simulink model "HW6_3"  (R2021a)
settings: Solver=VariableStepAuto  StartTime=0.0  StopTime=9  RelTol=1e-3
undefined symbols (not defined in the file or in its folder): w_fun
libraries: hdlBasic x207, simulink x2, xbsIndex_r4 x1
(part 1 of 2)
settings Model: Creator=hasith  LastModifiedBy=hasith

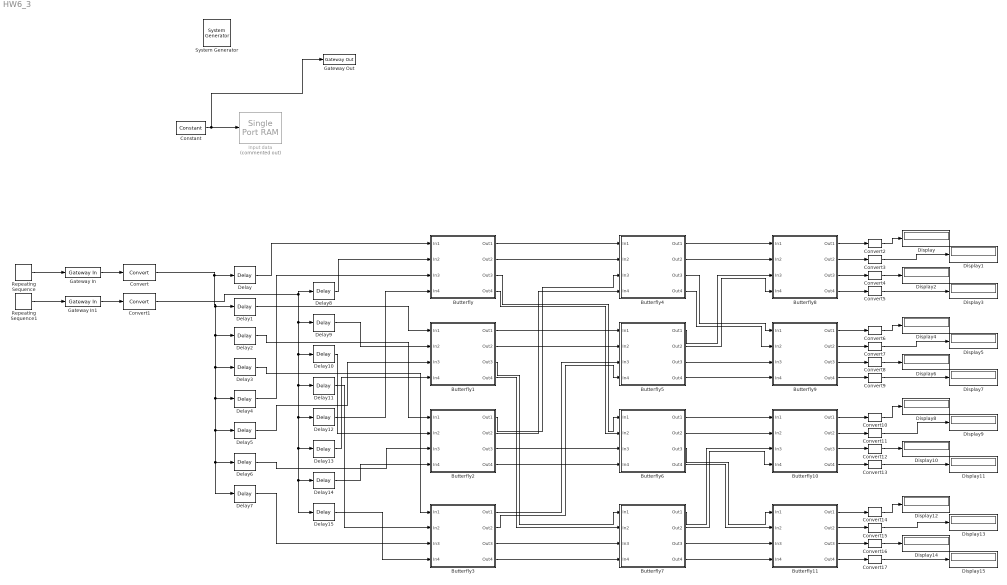
== system HW6_3 ==
  " System Generator" : xbsIndex_r4/ System Generator  Tag=genX  xilinxfamily=kintex7  part=xc7k325t  speed=-2  package=ffg900  synthesis_tool=Vivado  clock_wrapper=Clock Enables  directory=./netlist  proj_type=Vivado  Synth_file=Vivado Synthesis Defaults  Impl_file=Vivado Implementation Defaults  testbench=off  simulink_period=1  sysclk_period=10  dcm_input_clock_period=10  incr_netlist=off  trim_vbits=Everywhere in SubSystem  dbl_ovrd=According to Block Masks  core_generation=According to Block Masks  run_coregen=off  deprecated_control=off  eval_field=0  block_type=sysgen
  Butterfly : Subsystem  mask{wb_r=w_fun(0,8,1), wb_c=w_fun(0,8,1)}
      mask prompts: wb_r "w_r"; wb_c "w_c"
      mask Display:
      | port_label('input', 1, 'Re(x(n))')
      | port_label('input', 2, 'Im(x(n))')
      | port_label('input', 3, 'Re(x(n+N/2))')
      | port_label('input', 4, 'Im(x(n+N/2))')
      | 
      | 
      | port_label('output', 1, 'X_er')
      | port_label('output', 2, 'X_ei')
      | port_label('output', 3, 'X_or')
      | port_label('output',4, 'X_oi')
  Butterfly1 : Subsystem  mask{wb_r=w_fun(1,8,1), wb_c=w_fun(1,8,0)}
      mask prompts: wb_r "w_r"; wb_c "w_c"
      mask Display:
      | port_label('input', 1, 'Re(x(n))')
      | port_label('input', 2, 'Im(x(n))')
      | port_label('input', 3, 'Re(x(n+N/2))')
      | port_label('input', 4, 'Im(x(n+N/2))')
      | 
      | 
      | port_label('output', 1, 'X_er')
      | port_label('output', 2, 'X_ei')
      | port_label('output', 3, 'X_or')
      | port_label('output',4, 'X_oi')
  Butterfly10 : Subsystem  mask{wb_r=w_fun(0,8,1), wb_c=w_fun(0,8,0)}
      mask prompts: wb_r "w_r"; wb_c "w_c"
      mask Display:
      | port_label('input', 1, 'Re(x(n))')
      | port_label('input', 2, 'Im(x(n))')
      | port_label('input', 3, 'Re(x(n+N/2))')
      | port_label('input', 4, 'Im(x(n+N/2))')
      | 
      | 
      | port_label('output', 1, 'X_er')
      | port_label('output', 2, 'X_ei')
      | port_label('output', 3, 'X_or')
      | port_label('output',4, 'X_oi')
  Butterfly11 : Subsystem  mask{wb_r=w_fun(0,8,1), wb_c=w_fun(0,8,0)}
      mask prompts: wb_r "w_r"; wb_c "w_c"
      mask Display:
      | port_label('input', 1, 'Re(x(n))')
      | port_label('input', 2, 'Im(x(n))')
      | port_label('input', 3, 'Re(x(n+N/2))')
      | port_label('input', 4, 'Im(x(n+N/2))')
      | 
      | 
      | port_label('output', 1, 'X_er')
      | port_label('output', 2, 'X_ei')
      | port_label('output', 3, 'X_or')
      | port_label('output',4, 'X_oi')
  Butterfly2 : Subsystem  mask{wb_r=w_fun(2,8,1), wb_c=w_fun(2,8,0)}
      mask prompts: wb_r "w_r"; wb_c "w_c"
      mask Display:
      | port_label('input', 1, 'Re(x(n))')
      | port_label('input', 2, 'Im(x(n))')
      | port_label('input', 3, 'Re(x(n+N/2))')
      | port_label('input', 4, 'Im(x(n+N/2))')
      | 
      | 
      | port_label('output', 1, 'X_er')
      | port_label('output', 2, 'X_ei')
      | port_label('output', 3, 'X_or')
      | port_label('output',4, 'X_oi')
  Butterfly3 : Subsystem  mask{wb_r=w_fun(3,8,1), wb_c=w_fun(3,8,0)}
      mask prompts: wb_r "w_r"; wb_c "w_c"
      mask Display:
      | port_label('input', 1, 'Re(x(n))')
      | port_label('input', 2, 'Im(x(n))')
      | port_label('input', 3, 'Re(x(n+N/2))')
      | port_label('input', 4, 'Im(x(n+N/2))')
      | 
      | 
      | port_label('output', 1, 'X_er')
      | port_label('output', 2, 'X_ei')
      | port_label('output', 3, 'X_or')
      | port_label('output',4, 'X_oi')
  Butterfly4 : Subsystem  mask{wb_r=w_fun(0,8,1), wb_c=w_fun(0,8,0)}
      mask prompts: wb_r "w_r"; wb_c "w_c"
      mask Display:
      | port_label('input', 1, 'Re(x(n))')
      | port_label('input', 2, 'Im(x(n))')
      | port_label('input', 3, 'Re(x(n+N/2))')
      | port_label('input', 4, 'Im(x(n+N/2))')
      | 
      | 
      | port_label('output', 1, 'X_er')
      | port_label('output', 2, 'X_ei')
      | port_label('output', 3, 'X_or')
      | port_label('output',4, 'X_oi')
  Butterfly5 : Subsystem  mask{wb_r=w_fun(2,8,1), wb_c=w_fun(2,8,0)}
      mask prompts: wb_r "w_r"; wb_c "w_c"
      mask Display:
      | port_label('input', 1, 'Re(x(n))')
      | port_label('input', 2, 'Im(x(n))')
      | port_label('input', 3, 'Re(x(n+N/2))')
      | port_label('input', 4, 'Im(x(n+N/2))')
      | 
      | 
      | port_label('output', 1, 'X_er')
      | port_label('output', 2, 'X_ei')
      | port_label('output', 3, 'X_or')
      | port_label('output',4, 'X_oi')
  Butterfly6 : Subsystem  mask{wb_r=w_fun(0,8,1), wb_c=w_fun(0,8,0)}
      mask prompts: wb_r "w_r"; wb_c "w_c"
      mask Display:
      | port_label('input', 1, 'Re(x(n))')
      | port_label('input', 2, 'Im(x(n))')
      | port_label('input', 3, 'Re(x(n+N/2))')
      | port_label('input', 4, 'Im(x(n+N/2))')
      | 
      | 
      | port_label('output', 1, 'X_er')
      | port_label('output', 2, 'X_ei')
      | port_label('output', 3, 'X_or')
      | port_label('output',4, 'X_oi')
  Butterfly7 : Subsystem  mask{wb_r=w_fun(2,8,1), wb_c=w_fun(2,8,0)}
      mask prompts: wb_r "w_r"; wb_c "w_c"
      mask Display:
      | port_label('input', 1, 'Re(x(n))')
      | port_label('input', 2, 'Im(x(n))')
      | port_label('input', 3, 'Re(x(n+N/2))')
      | port_label('input', 4, 'Im(x(n+N/2))')
      | 
      | 
      | port_label('output', 1, 'X_er')
      | port_label('output', 2, 'X_ei')
      | port_label('output', 3, 'X_or')
      | port_label('output',4, 'X_oi')
  Butterfly8 : Subsystem  mask{wb_r=w_fun(0,8,1), wb_c=w_fun(0,8,0)}
      mask prompts: wb_r "w_r"; wb_c "w_c"
      mask Display:
      | port_label('input', 1, 'Re(x(n))')
      | port_label('input', 2, 'Im(x(n))')
      | port_label('input', 3, 'Re(x(n+N/2))')
      | port_label('input', 4, 'Im(x(n+N/2))')
      | 
      | 
      | port_label('output', 1, 'X_er')
      | port_label('output', 2, 'X_ei')
      | port_label('output', 3, 'X_or')
      | port_label('output',4, 'X_oi')
  Butterfly9 : Subsystem  mask{wb_r=w_fun(0,8,1), wb_c=w_fun(0,8,0)}
      mask prompts: wb_r "w_r"; wb_c "w_c"
      mask Display:
      | port_label('input', 1, 'Re(x(n))')
      | port_label('input', 2, 'Im(x(n))')
      | port_label('input', 3, 'Re(x(n+N/2))')
      | port_label('input', 4, 'Im(x(n+N/2))')
      | 
      | 
      | port_label('output', 1, 'X_er')
      | port_label('output', 2, 'X_ei')
      | port_label('output', 3, 'X_or')
      | port_label('output',4, 'X_oi')
  Constant : hdlBasic/Constant  const=0  gui_display_data_type=Fixed-point  arith_type=Signed (2's comp)  n_bits=8  bin_pt=0  preci_type=Custom  exp_width=9  frac_width=9  explicit_period=off  period=1  XmcBlockStatus=1  maskContainerNames=tabcontainer1  block_type=constant  block_config=sysgen:Constant_config
  Convert : hdlBasic/Convert  gui_display_data_type=Floating-point  arith_type=Floating-point  n_bits=16  bin_pt=14  float_type=Custom  exp_bits=9  fraction_bits=9  quantization=Truncate  overflow=Wrap  en=off  latency=0  pipeline=off  XmcBlockStatus=1  maskContainerNames=group2  block_type=convert  block_config=sysgen:Convert_config
  Convert1 : hdlBasic/Convert  gui_display_data_type=Floating-point  arith_type=Floating-point  n_bits=16  bin_pt=14  float_type=Custom  exp_bits=9  fraction_bits=9  quantization=Truncate  overflow=Wrap  en=off  latency=0  pipeline=off  XmcBlockStatus=1  maskContainerNames=group2  block_type=convert  block_config=sysgen:Convert_config
  Convert{2..17} (16 alike) : hdlBasic/Convert  gui_display_data_type=Floating-point  arith_type=Floating-point  n_bits=16  bin_pt=14  float_type=Single  exp_bits=9  fraction_bits=9  quantization=Truncate  overflow=Wrap  en=off  latency=0  pipeline=off  XmcBlockStatus=1  maskContainerNames=group2  block_type=convert  block_config=sysgen:Convert_config
  Delay : hdlBasic/Delay  rst=off  en=off  latency=1  reg_retiming=off  XmcBlockStatus=1  maskContainerNames=group1  block_type=delay  block_config=sysgen:Delay_config
  Delay1 : hdlBasic/Delay  rst=off  en=off  latency=2  reg_retiming=off  XmcBlockStatus=1  maskContainerNames=group1  block_type=delay  block_config=sysgen:Delay_config
  Delay10 : hdlBasic/Delay  rst=off  en=off  latency=3  reg_retiming=off  XmcBlockStatus=1  maskContainerNames=group1  block_type=delay  block_config=sysgen:Delay_config
  Delay11 : hdlBasic/Delay  rst=off  en=off  latency=4  reg_retiming=off  XmcBlockStatus=1  maskContainerNames=group1  block_type=delay  block_config=sysgen:Delay_config
  Delay12 : hdlBasic/Delay  rst=off  en=off  latency=5  reg_retiming=off  XmcBlockStatus=1  maskContainerNames=group1  block_type=delay  block_config=sysgen:Delay_config
  Delay13 : hdlBasic/Delay  rst=off  en=off  latency=6  reg_retiming=off  XmcBlockStatus=1  maskContainerNames=group1  block_type=delay  block_config=sysgen:Delay_config
  Delay14 : hdlBasic/Delay  rst=off  en=off  latency=7  reg_retiming=off  XmcBlockStatus=1  maskContainerNames=group1  block_type=delay  block_config=sysgen:Delay_config
  Delay15 : hdlBasic/Delay  rst=off  en=off  latency=8  reg_retiming=off  XmcBlockStatus=1  maskContainerNames=group1  block_type=delay  block_config=sysgen:Delay_config
  Delay2 : hdlBasic/Delay  rst=off  en=off  latency=3  reg_retiming=off  XmcBlockStatus=1  maskContainerNames=group1  block_type=delay  block_config=sysgen:Delay_config
  Delay3 : hdlBasic/Delay  rst=off  en=off  latency=4  reg_retiming=off  XmcBlockStatus=1  maskContainerNames=group1  block_type=delay  block_config=sysgen:Delay_config
  Delay4 : hdlBasic/Delay  rst=off  en=off  latency=5  reg_retiming=off  XmcBlockStatus=1  maskContainerNames=group1  block_type=delay  block_config=sysgen:Delay_config
  Delay5 : hdlBasic/Delay  rst=off  en=off  latency=6  reg_retiming=off  XmcBlockStatus=1  maskContainerNames=group1  block_type=delay  block_config=sysgen:Delay_config
  Delay6 : hdlBasic/Delay  rst=off  en=off  latency=7  reg_retiming=off  XmcBlockStatus=1  maskContainerNames=group1  block_type=delay  block_config=sysgen:Delay_config
  Delay7 : hdlBasic/Delay  rst=off  en=off  latency=8  reg_retiming=off  XmcBlockStatus=1  maskContainerNames=group1  block_type=delay  block_config=sysgen:Delay_config
  Delay8 : hdlBasic/Delay  rst=off  en=off  latency=1  reg_retiming=off  XmcBlockStatus=1  maskContainerNames=group1  block_type=delay  block_config=sysgen:Delay_config
  Delay9 : hdlBasic/Delay  rst=off  en=off  latency=2  reg_retiming=off  XmcBlockStatus=1  maskContainerNames=group1  block_type=delay  block_config=sysgen:Delay_config
  Display{,1..15} (16 alike) : Display
  Gateway In : hdlBasic/Gateway In  gui_display_data_type=Floating-point  arith_type=Floating-point  n_bits=8  bin_pt=0  preci_type=Single  exp_width=8  frac_width=24  rows=1  columns=1  quantization=Truncate  overflow=Saturate  period=1  UseAsADC=off  ADCChannel='1'  interface=None  automatic_assignment=on  address_offset=hex2dec('00')  intf_name=''  intf_description=''  default_value=0  timing_constraint=None  locs_specified=off  LOCs={}  io_standard={}  inherit_from_input=off  hdl_port=on  XmcBlockStatus=1  maskContainerNames=group4  block_type=gatewayin  block_config=sysgen:gateway_in_config  block_width_w=590  block_height_w=620  block_width=640  block_height=850
  Gateway In1 : hdlBasic/Gateway In  gui_display_data_type=Floating-point  arith_type=Floating-point  n_bits=8  bin_pt=0  preci_type=Single  exp_width=8  frac_width=24  rows=1  columns=1  quantization=Truncate  overflow=Saturate  period=1  UseAsADC=off  ADCChannel='1'  interface=None  automatic_assignment=on  address_offset=hex2dec('00')  intf_name=''  intf_description=''  default_value=0  timing_constraint=None  locs_specified=off  LOCs={}  io_standard={}  inherit_from_input=off  hdl_port=on  XmcBlockStatus=1  maskContainerNames=group4  block_type=gatewayin  block_config=sysgen:gateway_in_config  block_width_w=590  block_height_w=620  block_width=640  block_height=850
  Gateway Out : hdlBasic/Gateway Out  inherit_from_input=off  hdl_port=on  rows=1  columns=1  UseAsDAC=off  DACChannel='1'  interface=None  automatic_assignment=on  address_offset=hex2dec('00')  intf_name=''  intf_description=''  timing_constraint=None  locs_specified=off  LOCs={}  io_standard={}  XmcBlockStatus=1  maskContainerNames=group4  block_type=gatewayout  block_config=sysgen:gateway_out_config  block_width_w=590  block_height_w=620  block_width=620  block_height=750
  Input data : hdlBasic/Single Port RAM  Commented=on  depth=N  initVector=y  distributed_mem=Block RAM  write_mode=No Read On Write  rst=off  init_reg=0  en=off  optimize_latency=off  latency=1  optimize=Area  dbl_ovrd=off  simulation_type=fast_sim  XmcBlockStatus=1  maskContainerNames=tabcontainer1  block_type=spram  block_config=sysgen:SPRAM_config
  Repeating Sequence : simulink/Sources/Repeating Sequence  rep_seq_t=0:8  rep_seq_y=0:8
  Repeating Sequence1 : simulink/Sources/Repeating Sequence  rep_seq_t=0:8  rep_seq_y=[0 0 0 0 0 0 0 0 0]
  wires:
  Constant/1 -> Gateway Out/1, Input data/2
  Repeating Sequence/1 -> Gateway In/1
  Gateway In/1 -> Convert/1
  Gateway In1/1 -> Convert1/1
  Repeating Sequence1/1 -> Gateway In1/1
  Delay/1 -> Butterfly/1(In1)
  Delay8/1 -> Butterfly/2(In2)
  Delay4/1 -> Butterfly/3(In3)
  Delay12/1 -> Butterfly/4(In4)
  Delay9/1 -> Butterfly1/2(In2)
  Delay1/1 -> Butterfly1/1(In1)
  Delay5/1 -> Butterfly1/3(In3)
  Delay13/1 -> Butterfly1/4(In4)
  Delay2/1 -> Butterfly2/1(In1)
  Delay10/1 -> Butterfly2/2(In2)
  Delay6/1 -> Butterfly2/3(In3)
  Delay14/1 -> Butterfly2/4(In4)
  Delay3/1 -> Butterfly3/1(In1)
  Delay7/1 -> Butterfly3/3(In3)
  Delay11/1 -> Butterfly3/2(In2)
  Delay15/1 -> Butterfly3/4(In4)
  Butterfly/1(Out1) -> Butterfly4/1(In1)
  Butterfly/2(Out2) -> Butterfly4/2(In2)
  Butterfly2/1(Out1) -> Butterfly4/3(In3)
  Butterfly2/2(Out2) -> Butterfly4/4(In4)
  Butterfly1/1(Out1) -> Butterfly5/1(In1)
  Butterfly1/2(Out2) -> Butterfly5/2(In2)
  Butterfly3/1(Out1) -> Butterfly5/3(In3)
  Butterfly3/2(Out2) -> Butterfly5/4(In4)
  Butterfly/3(Out3) -> Butterfly6/1(In1)
  Butterfly/4(Out4) -> Butterfly6/2(In2)
  Butterfly2/3(Out3) -> Butterfly6/3(In3)
  Butterfly2/4(Out4) -> Butterfly6/4(In4)
  Butterfly1/3(Out3) -> Butterfly7/1(In1)
  Butterfly1/4(Out4) -> Butterfly7/2(In2)
  Butterfly3/3(Out3) -> Butterfly7/3(In3)
  Butterfly3/4(Out4) -> Butterfly7/4(In4)
  Butterfly4/1(Out1) -> Butterfly8/1(In1)
  Butterfly4/2(Out2) -> Butterfly8/2(In2)
  Butterfly5/1(Out1) -> Butterfly8/3(In3)
  Butterfly5/2(Out2) -> Butterfly8/4(In4)
  Butterfly4/3(Out3) -> Butterfly9/1(In1)
  Butterfly4/4(Out4) -> Butterfly9/2(In2)
  Butterfly5/3(Out3) -> Butterfly9/3(In3)
  Butterfly5/4(Out4) -> Butterfly9/4(In4)
  Butterfly6/1(Out1) -> Butterfly10/1(In1)
  Butterfly6/2(Out2) -> Butterfly10/2(In2)
  Butterfly7/4(Out4) -> Butterfly11/4(In4)
  Butterfly7/3(Out3) -> Butterfly11/3(In3)
  Butterfly6/3(Out3) -> Butterfly11/1(In1)
  Butterfly6/4(Out4) -> Butterfly11/2(In2)
  Butterfly7/1(Out1) -> Butterfly10/3(In3)
  Butterfly7/2(Out2) -> Butterfly10/4(In4)
  Convert/1 -> Delay2/1, Delay7/1, Delay6/1, Delay5/1, Delay4/1, Delay3/1, Delay1/1, Delay/1
  Convert1/1 -> Delay8/1, Delay11/1, Delay12/1, Delay15/1, Delay14/1, Delay13/1, Delay10/1, Delay9/1
  Butterfly8/1(Out1) -> Convert2/1
  Butterfly8/2(Out2) -> Convert3/1
  Butterfly8/3(Out3) -> Convert4/1
  Butterfly8/4(Out4) -> Convert5/1
  Convert2/1 -> Display/1
  Convert3/1 -> Display1/1
  Convert4/1 -> Display2/1
  Convert5/1 -> Display3/1
  Butterfly9/1(Out1) -> Convert6/1
  Butterfly9/2(Out2) -> Convert7/1
  Butterfly9/4(Out4) -> Convert9/1
  Convert6/1 -> Display4/1
  Butterfly9/3(Out3) -> Convert8/1
  Convert7/1 -> Display5/1
  Convert8/1 -> Display6/1
  Convert9/1 -> Display7/1
  Butterfly10/1(Out1) -> Convert10/1
  Butterfly10/2(Out2) -> Convert11/1
  Butterfly10/4(Out4) -> Convert13/1
  Convert10/1 -> Display8/1
  Butterfly10/3(Out3) -> Convert12/1
  Convert11/1 -> Display9/1
  Convert12/1 -> Display10/1
  Convert13/1 -> Display11/1
  Butterfly11/1(Out1) -> Convert14/1
  Butterfly11/2(Out2) -> Convert15/1
  Butterfly11/4(Out4) -> Convert17/1
  Convert14/1 -> Display12/1
  Butterfly11/3(Out3) -> Convert16/1
  Convert15/1 -> Display13/1
  Convert16/1 -> Display14/1
  Convert17/1 -> Display15/1

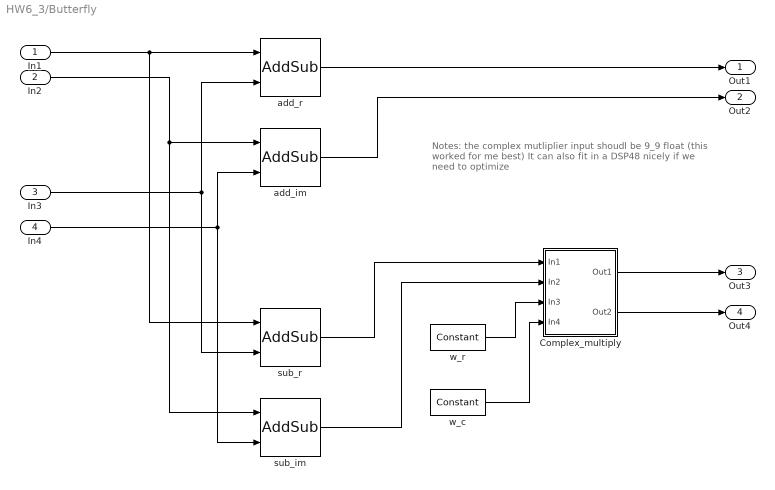
== system HW6_3/Butterfly ==
  note: Notes: the complex mutliplier
      | input shoudl be 9_9 float (this worked for me best)
      | It can also fit in a DSP48 nicely if we need to optimize
  In1 : Inport
  In2 : Inport  Port=2
  In3 : Inport  Port=3
  In4 : Inport  Port=4
  Complex_multiply : Subsystem
      mask Display:
      | port_label('input', 1, 'A')
      | port_label('input', 2, 'B')
      | port_label('input', 3, 'C')
      | port_label('input', 4, 'D')
      | 
      | 
      | port_label('output', 1, 'Real')
      | port_label('output', 2, 'Imag')
  add_im : hdlBasic/AddSub  mode=Addition  use_carryin=off  use_carryout=off  en=off  latency=0  precision=Full  arith_type=Unsigned  n_bits=16  bin_pt=14  quantization=Truncate  overflow=Wrap  use_behavioral_HDL=off  hw_selection=Fabric  pipelined=off  XmcBlockStatus=1  maskContainerNames=tabcontainer1  block_type=addsub  block_config=sysgen:Addsub_config
  add_r : hdlBasic/AddSub  mode=Addition  use_carryin=off  use_carryout=off  en=off  latency=0  precision=Full  arith_type=Unsigned  n_bits=16  bin_pt=14  quantization=Truncate  overflow=Wrap  use_behavioral_HDL=off  hw_selection=Fabric  pipelined=off  XmcBlockStatus=1  maskContainerNames=tabcontainer1  block_type=addsub  block_config=sysgen:Addsub_config
  sub_im : hdlBasic/AddSub  mode=Subtraction  use_carryin=off  use_carryout=off  en=off  latency=0  precision=Full  arith_type=Unsigned  n_bits=16  bin_pt=14  quantization=Truncate  overflow=Wrap  use_behavioral_HDL=off  hw_selection=Fabric  pipelined=off  XmcBlockStatus=1  maskContainerNames=tabcontainer1  block_type=addsub  block_config=sysgen:Addsub_config
  sub_r : hdlBasic/AddSub  mode=Subtraction  use_carryin=off  use_carryout=off  en=off  latency=0  precision=Full  arith_type=Unsigned  n_bits=16  bin_pt=14  quantization=Truncate  overflow=Wrap  use_behavioral_HDL=off  hw_selection=Fabric  pipelined=off  XmcBlockStatus=1  maskContainerNames=tabcontainer1  block_type=addsub  block_config=sysgen:Addsub_config
  w_c : hdlBasic/Constant  const=wb_c  gui_display_data_type=Floating-point  arith_type=Floating-point  n_bits=16  bin_pt=14  preci_type=Custom  exp_width=9  frac_width=9  explicit_period=off  period=1  XmcBlockStatus=1  maskContainerNames=tabcontainer1  block_type=constant  block_config=sysgen:Constant_config
  w_r : hdlBasic/Constant  const=wb_r  gui_display_data_type=Floating-point  arith_type=Floating-point  n_bits=16  bin_pt=14  preci_type=Custom  exp_width=9  frac_width=9  explicit_period=off  period=1  XmcBlockStatus=1  maskContainerNames=tabcontainer1  block_type=constant  block_config=sysgen:Constant_config
  Out1 : Outport
  Out2 : Outport  Port=2
  Out3 : Outport  Port=3
  Out4 : Outport  Port=4
  wires:
  Complex_multiply/2(Out2) -> Out4/1
  add_im/1 -> Out2/1
  w_r/1 -> Complex_multiply/3(In3)
  sub_r/1 -> Complex_multiply/1(In1)
  Complex_multiply/1(Out1) -> Out3/1
  In4/1 -> add_im/2, sub_im/2
  In3/1 -> add_r/2, sub_r/2
  add_r/1 -> Out1/1
  w_c/1 -> Complex_multiply/4(In4)
  sub_im/1 -> Complex_multiply/2(In2)
  In2/1 -> sub_im/1, add_im/1
  In1/1 -> sub_r/1, add_r/1

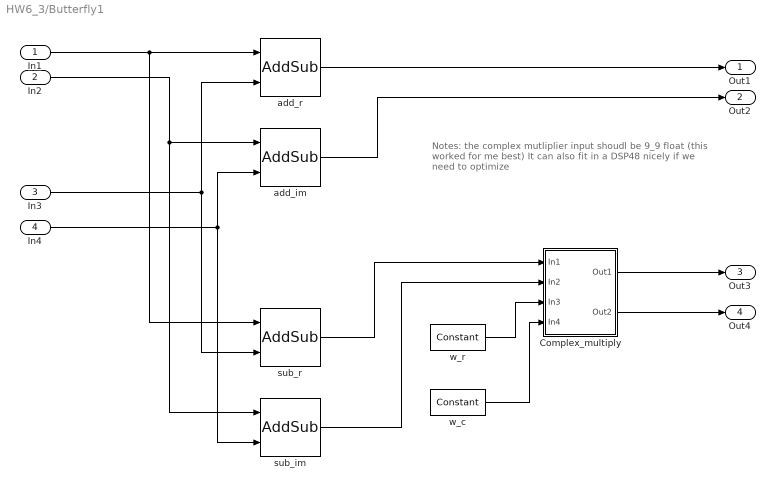
== system HW6_3/Butterfly1 ==
  note: Notes: the complex mutliplier
      | input shoudl be 9_9 float (this worked for me best)
      | It can also fit in a DSP48 nicely if we need to optimize
  In1 : Inport
  In2 : Inport  Port=2
  In3 : Inport  Port=3
  In4 : Inport  Port=4
  Complex_multiply : Subsystem
      mask Display:
      | port_label('input', 1, 'A')
      | port_label('input', 2, 'B')
      | port_label('input', 3, 'C')
      | port_label('input', 4, 'D')
      | 
      | 
      | port_label('output', 1, 'Real')
      | port_label('output', 2, 'Imag')
  add_im : hdlBasic/AddSub  mode=Addition  use_carryin=off  use_carryout=off  en=off  latency=0  precision=Full  arith_type=Unsigned  n_bits=16  bin_pt=14  quantization=Truncate  overflow=Wrap  use_behavioral_HDL=off  hw_selection=Fabric  pipelined=off  XmcBlockStatus=1  maskContainerNames=tabcontainer1  block_type=addsub  block_config=sysgen:Addsub_config
  add_r : hdlBasic/AddSub  mode=Addition  use_carryin=off  use_carryout=off  en=off  latency=0  precision=Full  arith_type=Unsigned  n_bits=16  bin_pt=14  quantization=Truncate  overflow=Wrap  use_behavioral_HDL=off  hw_selection=Fabric  pipelined=off  XmcBlockStatus=1  maskContainerNames=tabcontainer1  block_type=addsub  block_config=sysgen:Addsub_config
  sub_im : hdlBasic/AddSub  mode=Subtraction  use_carryin=off  use_carryout=off  en=off  latency=0  precision=Full  arith_type=Unsigned  n_bits=16  bin_pt=14  quantization=Truncate  overflow=Wrap  use_behavioral_HDL=off  hw_selection=Fabric  pipelined=off  XmcBlockStatus=1  maskContainerNames=tabcontainer1  block_type=addsub  block_config=sysgen:Addsub_config
  sub_r : hdlBasic/AddSub  mode=Subtraction  use_carryin=off  use_carryout=off  en=off  latency=0  precision=Full  arith_type=Unsigned  n_bits=16  bin_pt=14  quantization=Truncate  overflow=Wrap  use_behavioral_HDL=off  hw_selection=Fabric  pipelined=off  XmcBlockStatus=1  maskContainerNames=tabcontainer1  block_type=addsub  block_config=sysgen:Addsub_config
  w_c : hdlBasic/Constant  const=wb_c  gui_display_data_type=Floating-point  arith_type=Floating-point  n_bits=16  bin_pt=14  preci_type=Custom  exp_width=9  frac_width=9  explicit_period=off  period=1  XmcBlockStatus=1  maskContainerNames=tabcontainer1  block_type=constant  block_config=sysgen:Constant_config
  w_r : hdlBasic/Constant  const=wb_r  gui_display_data_type=Floating-point  arith_type=Floating-point  n_bits=16  bin_pt=14  preci_type=Custom  exp_width=9  frac_width=9  explicit_period=off  period=1  XmcBlockStatus=1  maskContainerNames=tabcontainer1  block_type=constant  block_config=sysgen:Constant_config
  Out1 : Outport
  Out2 : Outport  Port=2
  Out3 : Outport  Port=3
  Out4 : Outport  Port=4
  wires:
  Complex_multiply/2(Out2) -> Out4/1
  add_im/1 -> Out2/1
  w_r/1 -> Complex_multiply/3(In3)
  sub_r/1 -> Complex_multiply/1(In1)
  Complex_multiply/1(Out1) -> Out3/1
  In4/1 -> add_im/2, sub_im/2
  In3/1 -> add_r/2, sub_r/2
  add_r/1 -> Out1/1
  w_c/1 -> Complex_multiply/4(In4)
  sub_im/1 -> Complex_multiply/2(In2)
  In2/1 -> sub_im/1, add_im/1
  In1/1 -> sub_r/1, add_r/1

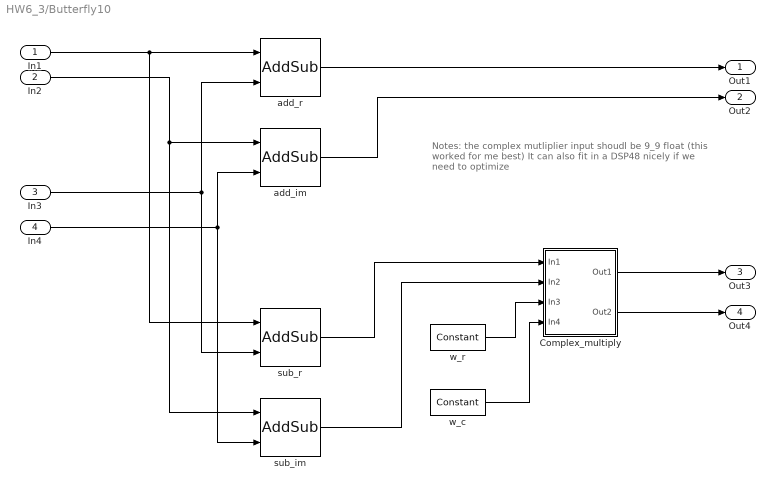
== system HW6_3/Butterfly10 ==
  note: Notes: the complex mutliplier
      | input shoudl be 9_9 float (this worked for me best)
      | It can also fit in a DSP48 nicely if we need to optimize
  In1 : Inport
  In2 : Inport  Port=2
  In3 : Inport  Port=3
  In4 : Inport  Port=4
  Complex_multiply : Subsystem
      mask Display:
      | port_label('input', 1, 'A')
      | port_label('input', 2, 'B')
      | port_label('input', 3, 'C')
      | port_label('input', 4, 'D')
      | 
      | 
      | port_label('output', 1, 'Real')
      | port_label('output', 2, 'Imag')
  add_im : hdlBasic/AddSub  mode=Addition  use_carryin=off  use_carryout=off  en=off  latency=0  precision=Full  arith_type=Unsigned  n_bits=16  bin_pt=14  quantization=Truncate  overflow=Wrap  use_behavioral_HDL=off  hw_selection=Fabric  pipelined=off  XmcBlockStatus=1  maskContainerNames=tabcontainer1  block_type=addsub  block_config=sysgen:Addsub_config
  add_r : hdlBasic/AddSub  mode=Addition  use_carryin=off  use_carryout=off  en=off  latency=0  precision=Full  arith_type=Unsigned  n_bits=16  bin_pt=14  quantization=Truncate  overflow=Wrap  use_behavioral_HDL=off  hw_selection=Fabric  pipelined=off  XmcBlockStatus=1  maskContainerNames=tabcontainer1  block_type=addsub  block_config=sysgen:Addsub_config
  sub_im : hdlBasic/AddSub  mode=Subtraction  use_carryin=off  use_carryout=off  en=off  latency=0  precision=Full  arith_type=Unsigned  n_bits=16  bin_pt=14  quantization=Truncate  overflow=Wrap  use_behavioral_HDL=off  hw_selection=Fabric  pipelined=off  XmcBlockStatus=1  maskContainerNames=tabcontainer1  block_type=addsub  block_config=sysgen:Addsub_config
  sub_r : hdlBasic/AddSub  mode=Subtraction  use_carryin=off  use_carryout=off  en=off  latency=0  precision=Full  arith_type=Unsigned  n_bits=16  bin_pt=14  quantization=Truncate  overflow=Wrap  use_behavioral_HDL=off  hw_selection=Fabric  pipelined=off  XmcBlockStatus=1  maskContainerNames=tabcontainer1  block_type=addsub  block_config=sysgen:Addsub_config
  w_c : hdlBasic/Constant  const=wb_c  gui_display_data_type=Floating-point  arith_type=Floating-point  n_bits=16  bin_pt=14  preci_type=Custom  exp_width=9  frac_width=9  explicit_period=off  period=1  XmcBlockStatus=1  maskContainerNames=tabcontainer1  block_type=constant  block_config=sysgen:Constant_config
  w_r : hdlBasic/Constant  const=wb_r  gui_display_data_type=Floating-point  arith_type=Floating-point  n_bits=16  bin_pt=14  preci_type=Custom  exp_width=9  frac_width=9  explicit_period=off  period=1  XmcBlockStatus=1  maskContainerNames=tabcontainer1  block_type=constant  block_config=sysgen:Constant_config
  Out1 : Outport
  Out2 : Outport  Port=2
  Out3 : Outport  Port=3
  Out4 : Outport  Port=4
  wires:
  Complex_multiply/2(Out2) -> Out4/1
  add_im/1 -> Out2/1
  w_r/1 -> Complex_multiply/3(In3)
  sub_r/1 -> Complex_multiply/1(In1)
  Complex_multiply/1(Out1) -> Out3/1
  In4/1 -> add_im/2, sub_im/2
  In3/1 -> add_r/2, sub_r/2
  add_r/1 -> Out1/1
  w_c/1 -> Complex_multiply/4(In4)
  sub_im/1 -> Complex_multiply/2(In2)
  In2/1 -> sub_im/1, add_im/1
  In1/1 -> sub_r/1, add_r/1

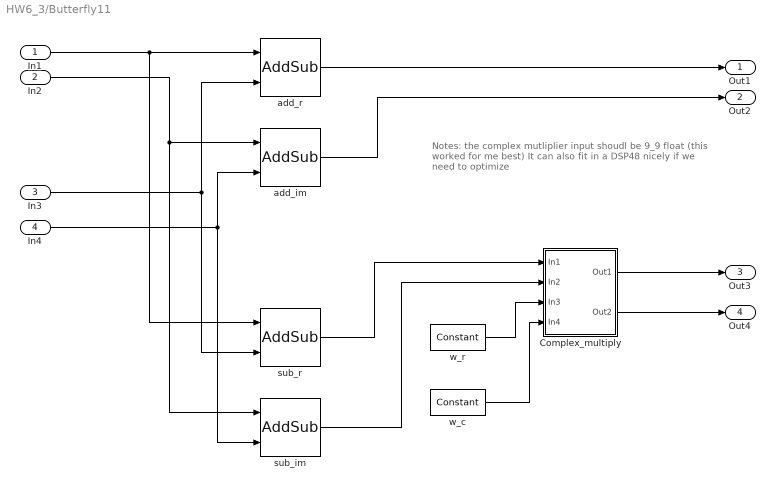
== system HW6_3/Butterfly11 ==
  note: Notes: the complex mutliplier
      | input shoudl be 9_9 float (this worked for me best)
      | It can also fit in a DSP48 nicely if we need to optimize
  In1 : Inport
  In2 : Inport  Port=2
  In3 : Inport  Port=3
  In4 : Inport  Port=4
  Complex_multiply : Subsystem
      mask Display:
      | port_label('input', 1, 'A')
      | port_label('input', 2, 'B')
      | port_label('input', 3, 'C')
      | port_label('input', 4, 'D')
      | 
      | 
      | port_label('output', 1, 'Real')
      | port_label('output', 2, 'Imag')
  add_im : hdlBasic/AddSub  mode=Addition  use_carryin=off  use_carryout=off  en=off  latency=0  precision=Full  arith_type=Unsigned  n_bits=16  bin_pt=14  quantization=Truncate  overflow=Wrap  use_behavioral_HDL=off  hw_selection=Fabric  pipelined=off  XmcBlockStatus=1  maskContainerNames=tabcontainer1  block_type=addsub  block_config=sysgen:Addsub_config
  add_r : hdlBasic/AddSub  mode=Addition  use_carryin=off  use_carryout=off  en=off  latency=0  precision=Full  arith_type=Unsigned  n_bits=16  bin_pt=14  quantization=Truncate  overflow=Wrap  use_behavioral_HDL=off  hw_selection=Fabric  pipelined=off  XmcBlockStatus=1  maskContainerNames=tabcontainer1  block_type=addsub  block_config=sysgen:Addsub_config
  sub_im : hdlBasic/AddSub  mode=Subtraction  use_carryin=off  use_carryout=off  en=off  latency=0  precision=Full  arith_type=Unsigned  n_bits=16  bin_pt=14  quantization=Truncate  overflow=Wrap  use_behavioral_HDL=off  hw_selection=Fabric  pipelined=off  XmcBlockStatus=1  maskContainerNames=tabcontainer1  block_type=addsub  block_config=sysgen:Addsub_config
  sub_r : hdlBasic/AddSub  mode=Subtraction  use_carryin=off  use_carryout=off  en=off  latency=0  precision=Full  arith_type=Unsigned  n_bits=16  bin_pt=14  quantization=Truncate  overflow=Wrap  use_behavioral_HDL=off  hw_selection=Fabric  pipelined=off  XmcBlockStatus=1  maskContainerNames=tabcontainer1  block_type=addsub  block_config=sysgen:Addsub_config
  w_c : hdlBasic/Constant  const=wb_c  gui_display_data_type=Floating-point  arith_type=Floating-point  n_bits=16  bin_pt=14  preci_type=Custom  exp_width=9  frac_width=9  explicit_period=off  period=1  XmcBlockStatus=1  maskContainerNames=tabcontainer1  block_type=constant  block_config=sysgen:Constant_config
  w_r : hdlBasic/Constant  const=wb_r  gui_display_data_type=Floating-point  arith_type=Floating-point  n_bits=16  bin_pt=14  preci_type=Custom  exp_width=9  frac_width=9  explicit_period=off  period=1  XmcBlockStatus=1  maskContainerNames=tabcontainer1  block_type=constant  block_config=sysgen:Constant_config
  Out1 : Outport
  Out2 : Outport  Port=2
  Out3 : Outport  Port=3
  Out4 : Outport  Port=4
  wires:
  Complex_multiply/2(Out2) -> Out4/1
  add_im/1 -> Out2/1
  w_r/1 -> Complex_multiply/3(In3)
  sub_r/1 -> Complex_multiply/1(In1)
  Complex_multiply/1(Out1) -> Out3/1
  In4/1 -> add_im/2, sub_im/2
  In3/1 -> add_r/2, sub_r/2
  add_r/1 -> Out1/1
  w_c/1 -> Complex_multiply/4(In4)
  sub_im/1 -> Complex_multiply/2(In2)
  In2/1 -> sub_im/1, add_im/1
  In1/1 -> sub_r/1, add_r/1

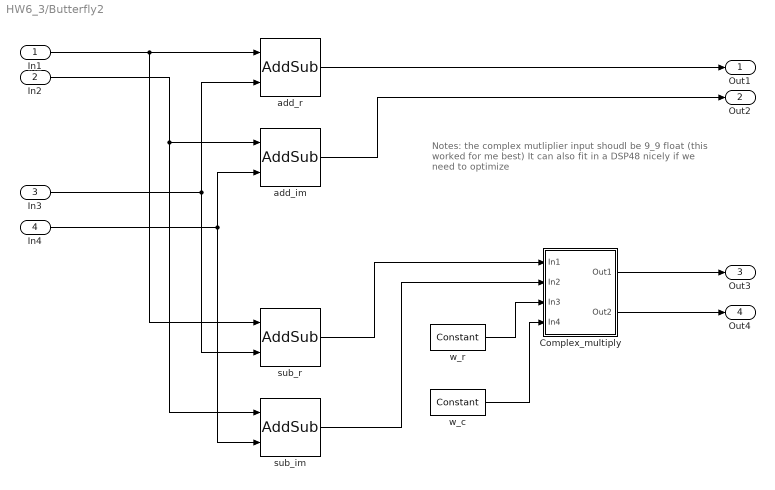
== system HW6_3/Butterfly2 ==
  note: Notes: the complex mutliplier
      | input shoudl be 9_9 float (this worked for me best)
      | It can also fit in a DSP48 nicely if we need to optimize
  In1 : Inport
  In2 : Inport  Port=2
  In3 : Inport  Port=3
  In4 : Inport  Port=4
  Complex_multiply : Subsystem
      mask Display:
      | port_label('input', 1, 'A')
      | port_label('input', 2, 'B')
      | port_label('input', 3, 'C')
      | port_label('input', 4, 'D')
      | 
      | 
      | port_label('output', 1, 'Real')
      | port_label('output', 2, 'Imag')
  add_im : hdlBasic/AddSub  mode=Addition  use_carryin=off  use_carryout=off  en=off  latency=0  precision=Full  arith_type=Unsigned  n_bits=16  bin_pt=14  quantization=Truncate  overflow=Wrap  use_behavioral_HDL=off  hw_selection=Fabric  pipelined=off  XmcBlockStatus=1  maskContainerNames=tabcontainer1  block_type=addsub  block_config=sysgen:Addsub_config
  add_r : hdlBasic/AddSub  mode=Addition  use_carryin=off  use_carryout=off  en=off  latency=0  precision=Full  arith_type=Unsigned  n_bits=16  bin_pt=14  quantization=Truncate  overflow=Wrap  use_behavioral_HDL=off  hw_selection=Fabric  pipelined=off  XmcBlockStatus=1  maskContainerNames=tabcontainer1  block_type=addsub  block_config=sysgen:Addsub_config
  sub_im : hdlBasic/AddSub  mode=Subtraction  use_carryin=off  use_carryout=off  en=off  latency=0  precision=Full  arith_type=Unsigned  n_bits=16  bin_pt=14  quantization=Truncate  overflow=Wrap  use_behavioral_HDL=off  hw_selection=Fabric  pipelined=off  XmcBlockStatus=1  maskContainerNames=tabcontainer1  block_type=addsub  block_config=sysgen:Addsub_config
  sub_r : hdlBasic/AddSub  mode=Subtraction  use_carryin=off  use_carryout=off  en=off  latency=0  precision=Full  arith_type=Unsigned  n_bits=16  bin_pt=14  quantization=Truncate  overflow=Wrap  use_behavioral_HDL=off  hw_selection=Fabric  pipelined=off  XmcBlockStatus=1  maskContainerNames=tabcontainer1  block_type=addsub  block_config=sysgen:Addsub_config
  w_c : hdlBasic/Constant  const=wb_c  gui_display_data_type=Floating-point  arith_type=Floating-point  n_bits=16  bin_pt=14  preci_type=Custom  exp_width=9  frac_width=9  explicit_period=off  period=1  XmcBlockStatus=1  maskContainerNames=tabcontainer1  block_type=constant  block_config=sysgen:Constant_config
  w_r : hdlBasic/Constant  const=wb_r  gui_display_data_type=Floating-point  arith_type=Floating-point  n_bits=16  bin_pt=14  preci_type=Custom  exp_width=9  frac_width=9  explicit_period=off  period=1  XmcBlockStatus=1  maskContainerNames=tabcontainer1  block_type=constant  block_config=sysgen:Constant_config
  Out1 : Outport
  Out2 : Outport  Port=2
  Out3 : Outport  Port=3
  Out4 : Outport  Port=4
  wires:
  Complex_multiply/2(Out2) -> Out4/1
  add_im/1 -> Out2/1
  w_r/1 -> Complex_multiply/3(In3)
  sub_r/1 -> Complex_multiply/1(In1)
  Complex_multiply/1(Out1) -> Out3/1
  In4/1 -> add_im/2, sub_im/2
  In3/1 -> add_r/2, sub_r/2
  add_r/1 -> Out1/1
  w_c/1 -> Complex_multiply/4(In4)
  sub_im/1 -> Complex_multiply/2(In2)
  In2/1 -> sub_im/1, add_im/1
  In1/1 -> sub_r/1, add_r/1

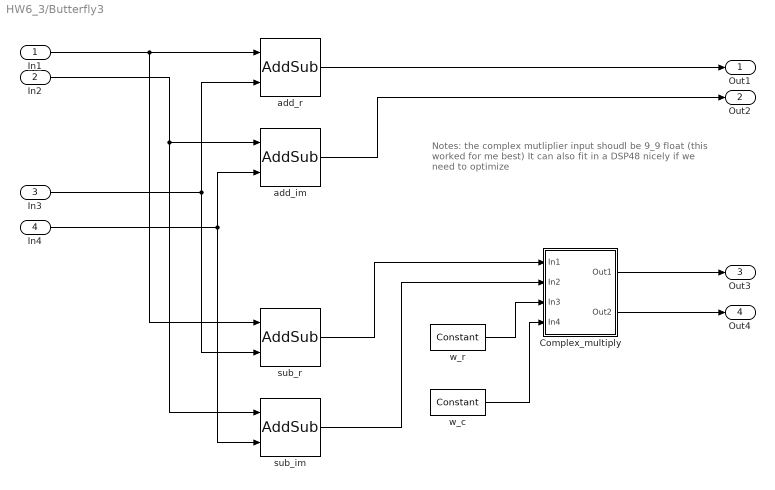
== system HW6_3/Butterfly3 ==
  note: Notes: the complex mutliplier
      | input shoudl be 9_9 float (this worked for me best)
      | It can also fit in a DSP48 nicely if we need to optimize
  In1 : Inport
  In2 : Inport  Port=2
  In3 : Inport  Port=3
  In4 : Inport  Port=4
  Complex_multiply : Subsystem
      mask Display:
      | port_label('input', 1, 'A')
      | port_label('input', 2, 'B')
      | port_label('input', 3, 'C')
      | port_label('input', 4, 'D')
      | 
      | 
      | port_label('output', 1, 'Real')
      | port_label('output', 2, 'Imag')
  add_im : hdlBasic/AddSub  mode=Addition  use_carryin=off  use_carryout=off  en=off  latency=0  precision=Full  arith_type=Unsigned  n_bits=16  bin_pt=14  quantization=Truncate  overflow=Wrap  use_behavioral_HDL=off  hw_selection=Fabric  pipelined=off  XmcBlockStatus=1  maskContainerNames=tabcontainer1  block_type=addsub  block_config=sysgen:Addsub_config
  add_r : hdlBasic/AddSub  mode=Addition  use_carryin=off  use_carryout=off  en=off  latency=0  precision=Full  arith_type=Unsigned  n_bits=16  bin_pt=14  quantization=Truncate  overflow=Wrap  use_behavioral_HDL=off  hw_selection=Fabric  pipelined=off  XmcBlockStatus=1  maskContainerNames=tabcontainer1  block_type=addsub  block_config=sysgen:Addsub_config
  sub_im : hdlBasic/AddSub  mode=Subtraction  use_carryin=off  use_carryout=off  en=off  latency=0  precision=Full  arith_type=Unsigned  n_bits=16  bin_pt=14  quantization=Truncate  overflow=Wrap  use_behavioral_HDL=off  hw_selection=Fabric  pipelined=off  XmcBlockStatus=1  maskContainerNames=tabcontainer1  block_type=addsub  block_config=sysgen:Addsub_config
  sub_r : hdlBasic/AddSub  mode=Subtraction  use_carryin=off  use_carryout=off  en=off  latency=0  precision=Full  arith_type=Unsigned  n_bits=16  bin_pt=14  quantization=Truncate  overflow=Wrap  use_behavioral_HDL=off  hw_selection=Fabric  pipelined=off  XmcBlockStatus=1  maskContainerNames=tabcontainer1  block_type=addsub  block_config=sysgen:Addsub_config
  w_c : hdlBasic/Constant  const=wb_c  gui_display_data_type=Floating-point  arith_type=Floating-point  n_bits=16  bin_pt=14  preci_type=Custom  exp_width=9  frac_width=9  explicit_period=off  period=1  XmcBlockStatus=1  maskContainerNames=tabcontainer1  block_type=constant  block_config=sysgen:Constant_config
  w_r : hdlBasic/Constant  const=wb_r  gui_display_data_type=Floating-point  arith_type=Floating-point  n_bits=16  bin_pt=14  preci_type=Custom  exp_width=9  frac_width=9  explicit_period=off  period=1  XmcBlockStatus=1  maskContainerNames=tabcontainer1  block_type=constant  block_config=sysgen:Constant_config
  Out1 : Outport
  Out2 : Outport  Port=2
  Out3 : Outport  Port=3
  Out4 : Outport  Port=4
  wires:
  Complex_multiply/2(Out2) -> Out4/1
  add_im/1 -> Out2/1
  w_r/1 -> Complex_multiply/3(In3)
  sub_r/1 -> Complex_multiply/1(In1)
  Complex_multiply/1(Out1) -> Out3/1
  In4/1 -> add_im/2, sub_im/2
  In3/1 -> add_r/2, sub_r/2
  add_r/1 -> Out1/1
  w_c/1 -> Complex_multiply/4(In4)
  sub_im/1 -> Complex_multiply/2(In2)
  In2/1 -> sub_im/1, add_im/1
  In1/1 -> sub_r/1, add_r/1

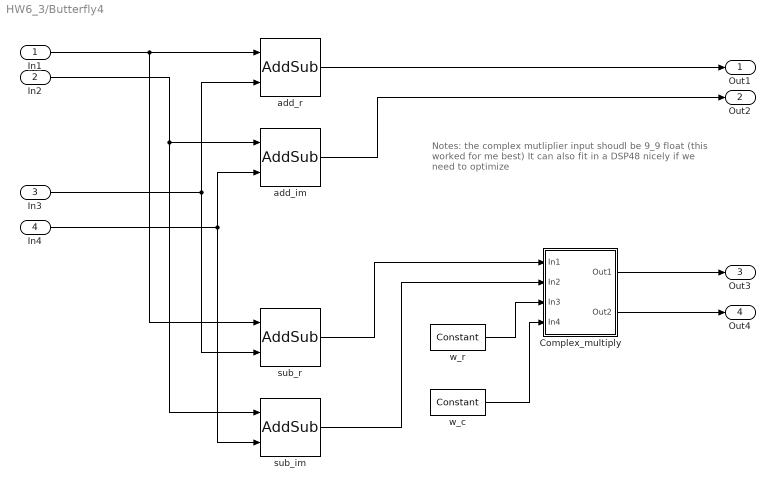
== system HW6_3/Butterfly4 ==
  note: Notes: the complex mutliplier
      | input shoudl be 9_9 float (this worked for me best)
      | It can also fit in a DSP48 nicely if we need to optimize
  In1 : Inport
  In2 : Inport  Port=2
  In3 : Inport  Port=3
  In4 : Inport  Port=4
  Complex_multiply : Subsystem
      mask Display:
      | port_label('input', 1, 'A')
      | port_label('input', 2, 'B')
      | port_label('input', 3, 'C')
      | port_label('input', 4, 'D')
      | 
      | 
      | port_label('output', 1, 'Real')
      | port_label('output', 2, 'Imag')
  add_im : hdlBasic/AddSub  mode=Addition  use_carryin=off  use_carryout=off  en=off  latency=0  precision=Full  arith_type=Unsigned  n_bits=16  bin_pt=14  quantization=Truncate  overflow=Wrap  use_behavioral_HDL=off  hw_selection=Fabric  pipelined=off  XmcBlockStatus=1  maskContainerNames=tabcontainer1  block_type=addsub  block_config=sysgen:Addsub_config
  add_r : hdlBasic/AddSub  mode=Addition  use_carryin=off  use_carryout=off  en=off  latency=0  precision=Full  arith_type=Unsigned  n_bits=16  bin_pt=14  quantization=Truncate  overflow=Wrap  use_behavioral_HDL=off  hw_selection=Fabric  pipelined=off  XmcBlockStatus=1  maskContainerNames=tabcontainer1  block_type=addsub  block_config=sysgen:Addsub_config
  sub_im : hdlBasic/AddSub  mode=Subtraction  use_carryin=off  use_carryout=off  en=off  latency=0  precision=Full  arith_type=Unsigned  n_bits=16  bin_pt=14  quantization=Truncate  overflow=Wrap  use_behavioral_HDL=off  hw_selection=Fabric  pipelined=off  XmcBlockStatus=1  maskContainerNames=tabcontainer1  block_type=addsub  block_config=sysgen:Addsub_config
  sub_r : hdlBasic/AddSub  mode=Subtraction  use_carryin=off  use_carryout=off  en=off  latency=0  precision=Full  arith_type=Unsigned  n_bits=16  bin_pt=14  quantization=Truncate  overflow=Wrap  use_behavioral_HDL=off  hw_selection=Fabric  pipelined=off  XmcBlockStatus=1  maskContainerNames=tabcontainer1  block_type=addsub  block_config=sysgen:Addsub_config
  w_c : hdlBasic/Constant  const=wb_c  gui_display_data_type=Floating-point  arith_type=Floating-point  n_bits=16  bin_pt=14  preci_type=Custom  exp_width=9  frac_width=9  explicit_period=off  period=1  XmcBlockStatus=1  maskContainerNames=tabcontainer1  block_type=constant  block_config=sysgen:Constant_config
  w_r : hdlBasic/Constant  const=wb_r  gui_display_data_type=Floating-point  arith_type=Floating-point  n_bits=16  bin_pt=14  preci_type=Custom  exp_width=9  frac_width=9  explicit_period=off  period=1  XmcBlockStatus=1  maskContainerNames=tabcontainer1  block_type=constant  block_config=sysgen:Constant_config
  Out1 : Outport
  Out2 : Outport  Port=2
  Out3 : Outport  Port=3
  Out4 : Outport  Port=4
  wires:
  Complex_multiply/2(Out2) -> Out4/1
  add_im/1 -> Out2/1
  w_r/1 -> Complex_multiply/3(In3)
  sub_r/1 -> Complex_multiply/1(In1)
  Complex_multiply/1(Out1) -> Out3/1
  In4/1 -> add_im/2, sub_im/2
  In3/1 -> add_r/2, sub_r/2
  add_r/1 -> Out1/1
  w_c/1 -> Complex_multiply/4(In4)
  sub_im/1 -> Complex_multiply/2(In2)
  In2/1 -> sub_im/1, add_im/1
  In1/1 -> sub_r/1, add_r/1

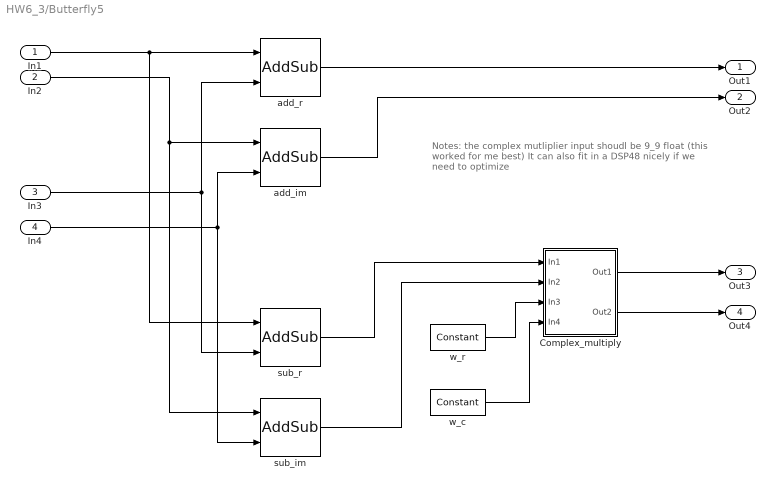
== system HW6_3/Butterfly5 ==
  note: Notes: the complex mutliplier
      | input shoudl be 9_9 float (this worked for me best)
      | It can also fit in a DSP48 nicely if we need to optimize
  In1 : Inport
  In2 : Inport  Port=2
  In3 : Inport  Port=3
  In4 : Inport  Port=4
  Complex_multiply : Subsystem
      mask Display:
      | port_label('input', 1, 'A')
      | port_label('input', 2, 'B')
      | port_label('input', 3, 'C')
      | port_label('input', 4, 'D')
      | 
      | 
      | port_label('output', 1, 'Real')
      | port_label('output', 2, 'Imag')
  add_im : hdlBasic/AddSub  mode=Addition  use_carryin=off  use_carryout=off  en=off  latency=0  precision=Full  arith_type=Unsigned  n_bits=16  bin_pt=14  quantization=Truncate  overflow=Wrap  use_behavioral_HDL=off  hw_selection=Fabric  pipelined=off  XmcBlockStatus=1  maskContainerNames=tabcontainer1  block_type=addsub  block_config=sysgen:Addsub_config
  add_r : hdlBasic/AddSub  mode=Addition  use_carryin=off  use_carryout=off  en=off  latency=0  precision=Full  arith_type=Unsigned  n_bits=16  bin_pt=14  quantization=Truncate  overflow=Wrap  use_behavioral_HDL=off  hw_selection=Fabric  pipelined=off  XmcBlockStatus=1  maskContainerNames=tabcontainer1  block_type=addsub  block_config=sysgen:Addsub_config
  sub_im : hdlBasic/AddSub  mode=Subtraction  use_carryin=off  use_carryout=off  en=off  latency=0  precision=Full  arith_type=Unsigned  n_bits=16  bin_pt=14  quantization=Truncate  overflow=Wrap  use_behavioral_HDL=off  hw_selection=Fabric  pipelined=off  XmcBlockStatus=1  maskContainerNames=tabcontainer1  block_type=addsub  block_config=sysgen:Addsub_config
  sub_r : hdlBasic/AddSub  mode=Subtraction  use_carryin=off  use_carryout=off  en=off  latency=0  precision=Full  arith_type=Unsigned  n_bits=16  bin_pt=14  quantization=Truncate  overflow=Wrap  use_behavioral_HDL=off  hw_selection=Fabric  pipelined=off  XmcBlockStatus=1  maskContainerNames=tabcontainer1  block_type=addsub  block_config=sysgen:Addsub_config
  w_c : hdlBasic/Constant  const=wb_c  gui_display_data_type=Floating-point  arith_type=Floating-point  n_bits=16  bin_pt=14  preci_type=Custom  exp_width=9  frac_width=9  explicit_period=off  period=1  XmcBlockStatus=1  maskContainerNames=tabcontainer1  block_type=constant  block_config=sysgen:Constant_config
  w_r : hdlBasic/Constant  const=wb_r  gui_display_data_type=Floating-point  arith_type=Floating-point  n_bits=16  bin_pt=14  preci_type=Custom  exp_width=9  frac_width=9  explicit_period=off  period=1  XmcBlockStatus=1  maskContainerNames=tabcontainer1  block_type=constant  block_config=sysgen:Constant_config
  Out1 : Outport
  Out2 : Outport  Port=2
  Out3 : Outport  Port=3
  Out4 : Outport  Port=4
  wires:
  Complex_multiply/2(Out2) -> Out4/1
  add_im/1 -> Out2/1
  w_r/1 -> Complex_multiply/3(In3)
  sub_r/1 -> Complex_multiply/1(In1)
  Complex_multiply/1(Out1) -> Out3/1
  In4/1 -> add_im/2, sub_im/2
  In3/1 -> add_r/2, sub_r/2
  add_r/1 -> Out1/1
  w_c/1 -> Complex_multiply/4(In4)
  sub_im/1 -> Complex_multiply/2(In2)
  In2/1 -> sub_im/1, add_im/1
  In1/1 -> sub_r/1, add_r/1

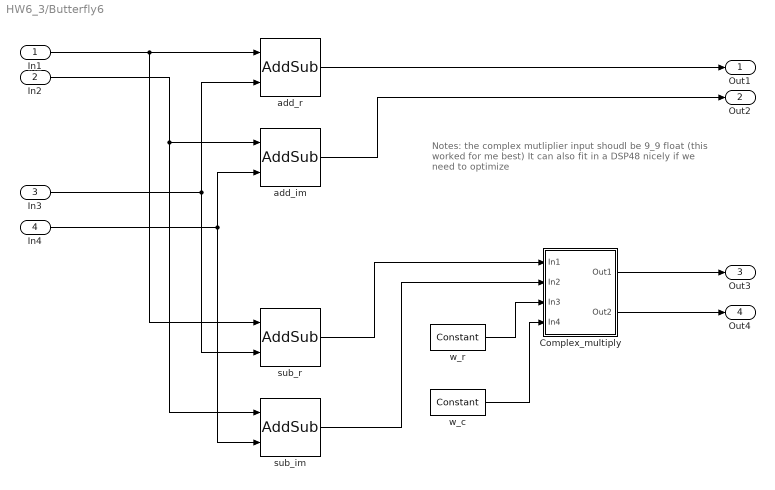
== system HW6_3/Butterfly6 ==
  note: Notes: the complex mutliplier
      | input shoudl be 9_9 float (this worked for me best)
      | It can also fit in a DSP48 nicely if we need to optimize
  In1 : Inport
  In2 : Inport  Port=2
  In3 : Inport  Port=3
  In4 : Inport  Port=4
  Complex_multiply : Subsystem
      mask Display:
      | port_label('input', 1, 'A')
      | port_label('input', 2, 'B')
      | port_label('input', 3, 'C')
      | port_label('input', 4, 'D')
      | 
      | 
      | port_label('output', 1, 'Real')
      | port_label('output', 2, 'Imag')
  add_im : hdlBasic/AddSub  mode=Addition  use_carryin=off  use_carryout=off  en=off  latency=0  precision=Full  arith_type=Unsigned  n_bits=16  bin_pt=14  quantization=Truncate  overflow=Wrap  use_behavioral_HDL=off  hw_selection=Fabric  pipelined=off  XmcBlockStatus=1  maskContainerNames=tabcontainer1  block_type=addsub  block_config=sysgen:Addsub_config
  add_r : hdlBasic/AddSub  mode=Addition  use_carryin=off  use_carryout=off  en=off  latency=0  precision=Full  arith_type=Unsigned  n_bits=16  bin_pt=14  quantization=Truncate  overflow=Wrap  use_behavioral_HDL=off  hw_selection=Fabric  pipelined=off  XmcBlockStatus=1  maskContainerNames=tabcontainer1  block_type=addsub  block_config=sysgen:Addsub_config
  sub_im : hdlBasic/AddSub  mode=Subtraction  use_carryin=off  use_carryout=off  en=off  latency=0  precision=Full  arith_type=Unsigned  n_bits=16  bin_pt=14  quantization=Truncate  overflow=Wrap  use_behavioral_HDL=off  hw_selection=Fabric  pipelined=off  XmcBlockStatus=1  maskContainerNames=tabcontainer1  block_type=addsub  block_config=sysgen:Addsub_config
  sub_r : hdlBasic/AddSub  mode=Subtraction  use_carryin=off  use_carryout=off  en=off  latency=0  precision=Full  arith_type=Unsigned  n_bits=16  bin_pt=14  quantization=Truncate  overflow=Wrap  use_behavioral_HDL=off  hw_selection=Fabric  pipelined=off  XmcBlockStatus=1  maskContainerNames=tabcontainer1  block_type=addsub  block_config=sysgen:Addsub_config
  w_c : hdlBasic/Constant  const=wb_c  gui_display_data_type=Floating-point  arith_type=Floating-point  n_bits=16  bin_pt=14  preci_type=Custom  exp_width=9  frac_width=9  explicit_period=off  period=1  XmcBlockStatus=1  maskContainerNames=tabcontainer1  block_type=constant  block_config=sysgen:Constant_config
  w_r : hdlBasic/Constant  const=wb_r  gui_display_data_type=Floating-point  arith_type=Floating-point  n_bits=16  bin_pt=14  preci_type=Custom  exp_width=9  frac_width=9  explicit_period=off  period=1  XmcBlockStatus=1  maskContainerNames=tabcontainer1  block_type=constant  block_config=sysgen:Constant_config
  Out1 : Outport
  Out2 : Outport  Port=2
  Out3 : Outport  Port=3
  Out4 : Outport  Port=4
  wires:
  Complex_multiply/2(Out2) -> Out4/1
  add_im/1 -> Out2/1
  w_r/1 -> Complex_multiply/3(In3)
  sub_r/1 -> Complex_multiply/1(In1)
  Complex_multiply/1(Out1) -> Out3/1
  In4/1 -> add_im/2, sub_im/2
  In3/1 -> add_r/2, sub_r/2
  add_r/1 -> Out1/1
  w_c/1 -> Complex_multiply/4(In4)
  sub_im/1 -> Complex_multiply/2(In2)
  In2/1 -> sub_im/1, add_im/1
  In1/1 -> sub_r/1, add_r/1

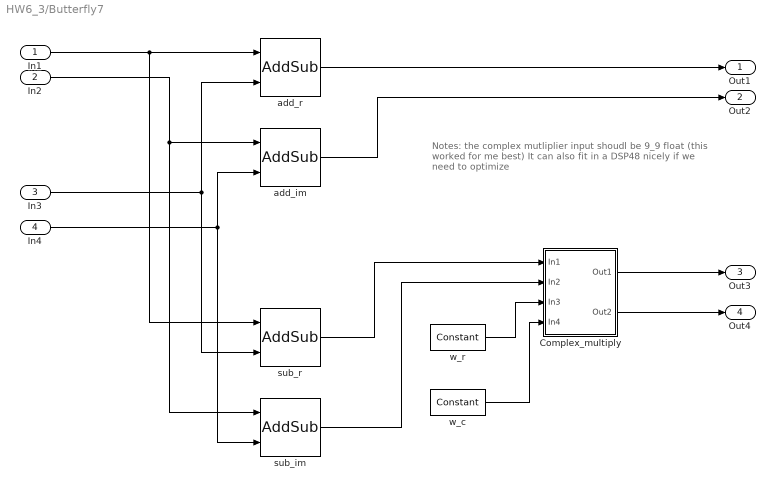
== system HW6_3/Butterfly7 ==
  note: Notes: the complex mutliplier
      | input shoudl be 9_9 float (this worked for me best)
      | It can also fit in a DSP48 nicely if we need to optimize
  In1 : Inport
  In2 : Inport  Port=2
  In3 : Inport  Port=3
  In4 : Inport  Port=4
  Complex_multiply : Subsystem
      mask Display:
      | port_label('input', 1, 'A')
      | port_label('input', 2, 'B')
      | port_label('input', 3, 'C')
      | port_label('input', 4, 'D')
      | 
      | 
      | port_label('output', 1, 'Real')
      | port_label('output', 2, 'Imag')
  add_im : hdlBasic/AddSub  mode=Addition  use_carryin=off  use_carryout=off  en=off  latency=0  precision=Full  arith_type=Unsigned  n_bits=16  bin_pt=14  quantization=Truncate  overflow=Wrap  use_behavioral_HDL=off  hw_selection=Fabric  pipelined=off  XmcBlockStatus=1  maskContainerNames=tabcontainer1  block_type=addsub  block_config=sysgen:Addsub_config
  add_r : hdlBasic/AddSub  mode=Addition  use_carryin=off  use_carryout=off  en=off  latency=0  precision=Full  arith_type=Unsigned  n_bits=16  bin_pt=14  quantization=Truncate  overflow=Wrap  use_behavioral_HDL=off  hw_selection=Fabric  pipelined=off  XmcBlockStatus=1  maskContainerNames=tabcontainer1  block_type=addsub  block_config=sysgen:Addsub_config
  sub_im : hdlBasic/AddSub  mode=Subtraction  use_carryin=off  use_carryout=off  en=off  latency=0  precision=Full  arith_type=Unsigned  n_bits=16  bin_pt=14  quantization=Truncate  overflow=Wrap  use_behavioral_HDL=off  hw_selection=Fabric  pipelined=off  XmcBlockStatus=1  maskContainerNames=tabcontainer1  block_type=addsub  block_config=sysgen:Addsub_config
  sub_r : hdlBasic/AddSub  mode=Subtraction  use_carryin=off  use_carryout=off  en=off  latency=0  precision=Full  arith_type=Unsigned  n_bits=16  bin_pt=14  quantization=Truncate  overflow=Wrap  use_behavioral_HDL=off  hw_selection=Fabric  pipelined=off  XmcBlockStatus=1  maskContainerNames=tabcontainer1  block_type=addsub  block_config=sysgen:Addsub_config
  w_c : hdlBasic/Constant  const=wb_c  gui_display_data_type=Floating-point  arith_type=Floating-point  n_bits=16  bin_pt=14  preci_type=Custom  exp_width=9  frac_width=9  explicit_period=off  period=1  XmcBlockStatus=1  maskContainerNames=tabcontainer1  block_type=constant  block_config=sysgen:Constant_config
  w_r : hdlBasic/Constant  const=wb_r  gui_display_data_type=Floating-point  arith_type=Floating-point  n_bits=16  bin_pt=14  preci_type=Custom  exp_width=9  frac_width=9  explicit_period=off  period=1  XmcBlockStatus=1  maskContainerNames=tabcontainer1  block_type=constant  block_config=sysgen:Constant_config
  Out1 : Outport
  Out2 : Outport  Port=2
  Out3 : Outport  Port=3
  Out4 : Outport  Port=4
  wires:
  Complex_multiply/2(Out2) -> Out4/1
  add_im/1 -> Out2/1
  w_r/1 -> Complex_multiply/3(In3)
  sub_r/1 -> Complex_multiply/1(In1)
  Complex_multiply/1(Out1) -> Out3/1
  In4/1 -> add_im/2, sub_im/2
  In3/1 -> add_r/2, sub_r/2
  add_r/1 -> Out1/1
  w_c/1 -> Complex_multiply/4(In4)
  sub_im/1 -> Complex_multiply/2(In2)
  In2/1 -> sub_im/1, add_im/1
  In1/1 -> sub_r/1, add_r/1
